simulink model "mcb_resolver_f28379d"  (R2026a)
settings: Solver=FixedStepDiscrete  StopTime=5  EnableMultiTasking=on
InitFcn:
  | mcb_resolver_f28379d_data;
values from neighbouring files (symbols this model uses):
  dataType = 'single'    [mcb_resolver_f28379d_data.m]
undefined symbols (not defined in the file or in its folder): resolver
libraries: simulink x5, c280xlib x2, c2837xDlib x2, svdutilitieslib x1
Description:
  | CN0276 AD2S1210 absolute-position monitor using GPIO29 SAMPLE and SPIA.
settings Model: ExtModeTrigDuration=8  Creator=The MathWorks, Inc.  LastModifiedBy=User
settings OptimizationCC: DefaultUnderspecifiedDataType=single  MaxStackSize=1024  DenormalBehavior=FlushToZero
settings DebuggingCC: MultiTaskDSMMsg=none  ParameterPrecisionLossMsg=none
settings HardwareCC: ProdBitPerChar=16.0  ProdBitPerInt=16.0  ProdLargestAtomicInteger=Integer  ProdWordSize=16.0  ProdHWDeviceType=Texas Instruments->C2000
settings RTWCC: SystemTargetFile=ert.tlc  HardwareBoard=TI Delfino F28379D LaunchPad  TLCOptions=-aInlineSetEventsForThisBaseRateFcn=TLC_FALSE -aSuppressMultiTaskScheduler=TLC_FALSE -aRateBasedStepFcn=1  GenerateReport=on  Toolchain=Texas Instruments Code Composer Studio (C2000)  IncludeHyperlinkInReport=on  GenerateTraceInfo=on  GenerateTraceReport=on  GenerateTraceReportSl=on  GenerateTraceReportSf=on  GenerateTraceReportEml=on  Description=Embedded Coder
settings ERTTargetCC: ExtModeStaticAllocSize=10000.0  DynamicArrayContainerType=coder::array  CodeReplacementLibrary=TI C28x

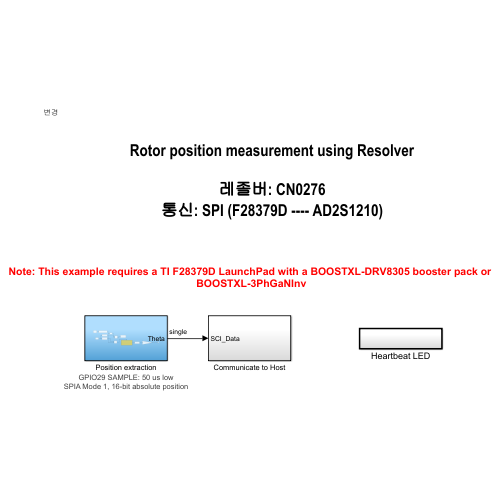
[thumbnail: Simulink's stored preview of the top-level diagram]
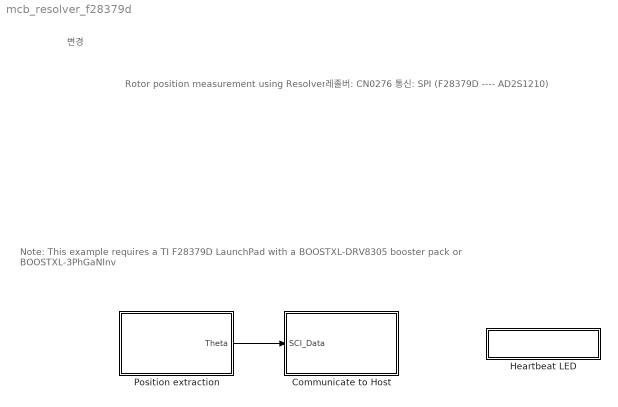
== system mcb_resolver_f28379d ==
  note: 변경
  note: Note: This example requires a TI F28379D LaunchPad with a BOOSTXL-DRV8305 booster pack or
      | BOOSTXL-3PhGaNInv
  note: Rotor position measurement using Resolver
      |
      | 레졸버: CN0276
      | 통신: SPI (F28379D ---- AD2S1210)
  Communicate to Host : Subsystem
  Heartbeat LED : Subsystem  TreatAsAtomicUnit=on
  Position extraction : Subsystem
      settings: AttributesFormatString=GPIO29 SAMPLE: 50 us low\nSPIA Mode 1, 16-bit absolute position
  wires:
  Position extraction/1(Theta) -> Communicate to Host/1(SCI_Data)

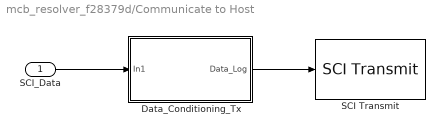
== system mcb_resolver_f28379d/Communicate to Host ==
  SCI_Data : Inport
  Data_Conditioning_Tx : Subsystem  Variant=on
  SCI Transmit : c280xlib/SCI Transmit  sciModule=A  dataHead='SS'  dataTail='EE'  frameSize=600  blockingMode=on  outputStatus=off
  wires:
  SCI_Data/1 -> Data_Conditioning_Tx/1(In1)
  Data_Conditioning_Tx/1(Data_Log) -> SCI Transmit/1

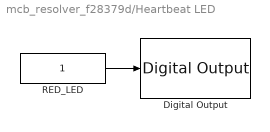
== system mcb_resolver_f28379d/Heartbeat LED ==
  Digital Output : c2837xDlib/Digital Output  GPIO_Number=GPIO32~GPIO39  GPIO_Bit0=off  GPIO_BIT0_Toggle=on  GPIO_Bit1=off  GPIO_BIT1_Toggle=off  GPIO_Bit2=on  GPIO_BIT2_Toggle=on  GPIO_Bit3=off  GPIO_BIT3_Toggle=off  GPIO_Bit4=off  GPIO_BIT4_Toggle=off  GPIO_Bit5=off  GPIO_BIT5_Toggle=off  GPIO_Bit6=off  GPIO_BIT6_Toggle=off  GPIO_Bit7=off  GPIO_BIT7_Toggle=off
  RED_LED : Constant  OutDataTypeStr=uint16  SampleTime=0.5
  wires:
  RED_LED/1 -> Digital Output/1

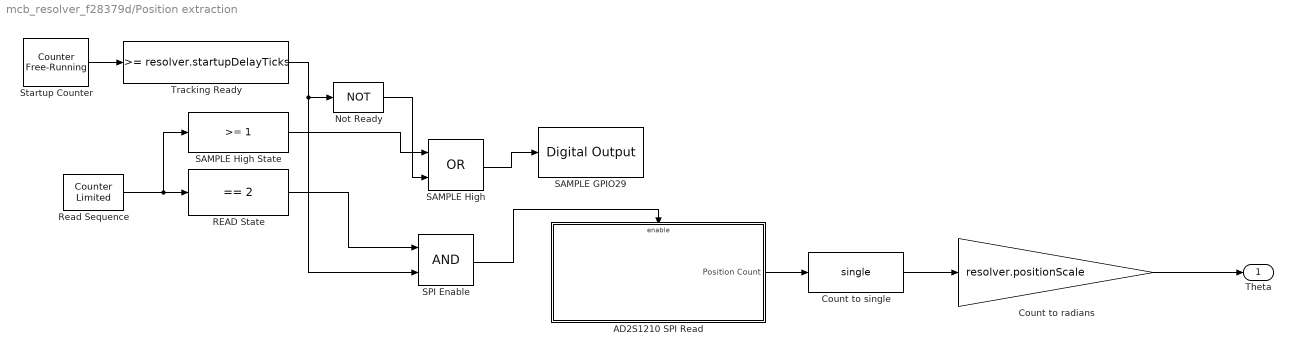
== system mcb_resolver_f28379d/Position extraction ==
  AD2S1210 SPI Read : Subsystem  TreatAsAtomicUnit=on
  Count to radians : Gain  Gain=resolver.positionScale  OutDataTypeStr=single
  Count to single : DataTypeConversion  OutDataTypeStr=single  SaturateOnIntegerOverflow=off  RndMeth=Floor
  Not Ready : Logic  Operator=NOT  Inputs=1  AllPortsSameDT=off  OutDataTypeStr=boolean
  READ State : simulink/Logic and Bit Operations/Compare To Constant  relop===  const=2  OutDataTypeStr=boolean  ZeroCross=off
  Read Sequence : simulink/Sources/Counter Limited  uplimit=2  tsamp=Ts
  SAMPLE GPIO29 : c2837xDlib/Digital Output  GPIO_Number=GPIO24~GPIO31  GPIO_Bit0=off  GPIO_BIT0_Toggle=off  GPIO_Bit1=off  GPIO_BIT1_Toggle=off  GPIO_Bit2=off  GPIO_BIT2_Toggle=off  GPIO_Bit3=off  GPIO_BIT3_Toggle=off  GPIO_Bit4=off  GPIO_BIT4_Toggle=off  GPIO_Bit5=on  GPIO_BIT5_Toggle=off  GPIO_Bit6=off  GPIO_BIT6_Toggle=off  GPIO_Bit7=off  GPIO_BIT7_Toggle=off
  SAMPLE High : Logic  Operator=OR  AllPortsSameDT=off  OutDataTypeStr=boolean
  SAMPLE High State : simulink/Logic and Bit Operations/Compare To Constant  relop=>=  const=1  OutDataTypeStr=boolean  ZeroCross=off
  SPI Enable : Logic  AllPortsSameDT=off  OutDataTypeStr=boolean
  Startup Counter : simulink/Sources/Counter Free-Running  NumBits=32  tsamp=Ts
  Tracking Ready : simulink/Logic and Bit Operations/Compare To Constant  relop=>=  const=resolver.startupDelayTicks  OutDataTypeStr=boolean  ZeroCross=off
  Theta : Outport  OutDataTypeStr=single
  wires:
  Startup Counter/1 -> Tracking Ready/1
  Tracking Ready/1 -> SPI Enable/2, Not Ready/1
  Read Sequence/1 -> READ State/1, SAMPLE High State/1
  READ State/1 -> SPI Enable/1
  Not Ready/1 -> SAMPLE High/2
  SAMPLE High/1 -> SAMPLE GPIO29/1
  SPI Enable/1 -> AD2S1210 SPI Read/Enable
  AD2S1210 SPI Read/1(Position Count) -> Count to single/1
  Count to single/1 -> Count to radians/1
  Count to radians/1 -> Theta/1
  SAMPLE High State/1 -> SAMPLE High/1

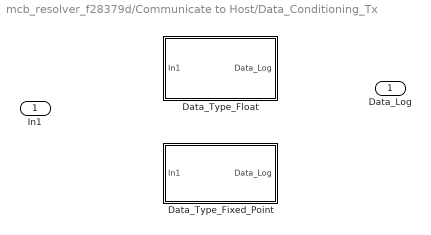
== system mcb_resolver_f28379d/Communicate to Host/Data_Conditioning_Tx ==
  In1 : Inport
  Data_Type_Fixed_Point : Subsystem  VariantControl=~isequal(dataType,'single')
  Data_Type_Float : Subsystem  VariantControl=isequal(dataType, 'single')
  Data_Log : Outport

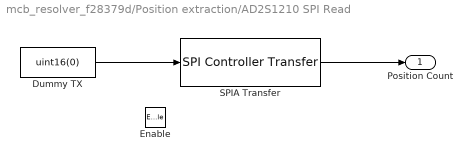
== system mcb_resolver_f28379d/Position extraction/AD2S1210 SPI Read ==
  Enable : EnablePort
  Dummy TX : Constant  Value=uint16(0)  OutDataTypeStr=uint16  SampleTime=-1
  SPIA Transfer : c280xlib/SPI Controller Transfer  SPISelect=SPI_A  ClockPolarity=Rising_edge  ClockPhase=Delay_half_cycle  SPIModule=uint32(0)  Mode=Master  BusSpeed=resolver.spiFrequency  FirstBitToTransfer=Most significant bit (MSB)  ClockMode=1  BlockFunction=Transfer  EnableRegisterAddress=off  RegisterAddress=0  OutputDataType=uint16  OutputDataLength=1  DataBits=16  UseCustomSSPin=Provided by the SPI peripheral  ActiveLowSSPin=Active low  Pin=61
  Position Count : Outport  OutDataTypeStr=uint16  InitialOutput=0
  wires:
  Dummy TX/1 -> SPIA Transfer/1
  SPIA Transfer/1 -> Position Count/1

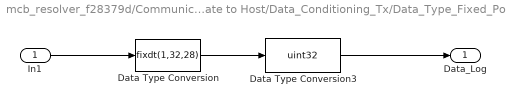
== system mcb_resolver_f28379d/Communicate to Host/Data_Conditioning_Tx/Data_Type_Fixed_Point ==
  In1 : Inport
  Data Type Conversion : DataTypeConversion  OutDataTypeStr=fixdt(1,32,28)  RndMeth=Simplest  SaturateOnIntegerOverflow=off
  Data Type Conversion3 : DataTypeConversion  OutDataTypeStr=uint32  ConvertRealWorld=Stored Integer (SI)  RndMeth=Simplest  SaturateOnIntegerOverflow=off
  Data_Log : Outport
  wires:
  In1/1 -> Data Type Conversion/1
  Data Type Conversion3/1 -> Data_Log/1
  Data Type Conversion/1 -> Data Type Conversion3/1

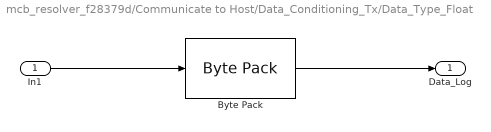
== system mcb_resolver_f28379d/Communicate to Host/Data_Conditioning_Tx/Data_Type_Float ==
  In1 : Inport
  Byte Pack : svdutilitieslib/Byte Pack  maskPackedDataType=uint32  datatypes={'single'}  byteAlign=4  blockPlatform=tic2000
  Data_Log : Outport
  wires:
  Byte Pack/1 -> Data_Log/1
  In1/1 -> Byte Pack/1
